simulink model "v2_4_debug3"  (R2017a)
settings: Solver=VariableStepAuto  StartTime=0.0  StopTime=50  RelTol=1e-3
values from neighbouring files (symbols this model uses):
  EbN0 = 6    [v2_4_debug1sI.m]    (also in v2_4_debug2sI.m; v2_4_debug3m.m; v2_4_randomm.m = 7; v2_4_randomm2.m)
  TracebackDepth = 64    [v2_4_debug1sI.m]    (also in v2_4_debug2sI.m; v2_4_debug3m.m; v2_4_randomm.m; v2_4_randomm2.m)
libraries: commblkintrlv2 x2, commchan3 x2, commdigbbndpm3 x1, commrandsrc3 x1, dspquant2 x1, commsink2 x1
settings Model: Creator=DELL  LastModifiedBy=DELL

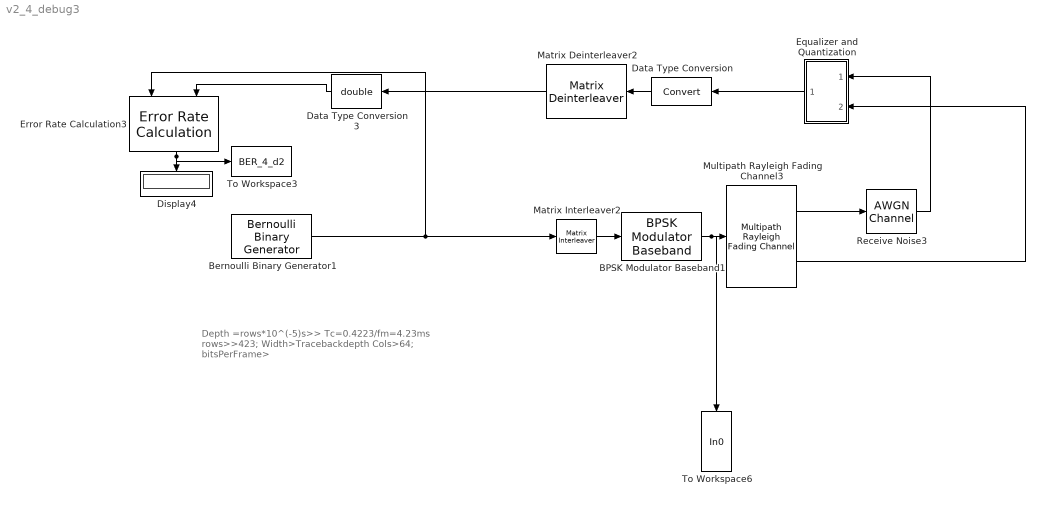
== system v2_4_debug3 ==
  note: Depth =rows*10^(-5)s>> Tc=0.4223/fm=4.23ms
      | 	rows>>423;
      |
      | Width>Tracebackdepth
      | 	Cols>64;
      |
      | bitsPerFrame>
  BPSK Modulator Baseband1 : commdigbbndpm3/BPSK Modulator Baseband  Ph=0  outDtype=double  outWordLen=16  outUDDataType=sfix(16)  outFracLenMode=Best precision  outFracLen=15  outDataTypeStr=double  outLastDataTypeStr=double
  Bernoulli Binary Generator1 : commrandsrc3/Bernoulli Binary Generator  ProbabilityOfZero=0.5  SeedSource=Auto  Seed=0  SampleTime=1e-5  SamplesPerFrame=SamplesPerFrame  OutputDataType=double  SimulateUsing=Interpreted execution
  Data Type Conversion : DataTypeConversion  SaturateOnIntegerOverflow=on  RndMeth=Zero
  Data Type Conversion3 : DataTypeConversion  OutDataTypeStr=double
  Display4 : Display
  Equalizer and Quantization : Subsystem
  Error Rate Calculation3 : commsink2/Error Rate Calculation  N=TracebackDepth  st_delay=0  cp_mode=Entire frame  subframe=[]  PMode=Port  WsName=ErrorVec  RsMode2=off  stop=off  numErr=100  maxBits=1e6
  Matrix Deinterleaver2 : commblkintrlv2/Matrix Deinterleaver  Nrows=Rows  Ncols=Cols
      settings: SourceProductName=Communications System Toolbox  SourceProductBaseCode=CM
  Matrix Interleaver2 : commblkintrlv2/Matrix Interleaver  Nrows=Rows  Ncols=Cols
      settings: SourceProductName=Communications System Toolbox  SourceProductBaseCode=CM
  Multipath Rayleigh Fading Channel3 : commchan3/Multipath Rayleigh Fading Channel  maxDopplerShift=100  spectrumType=Jakes  sigmaGaussian=1/sqrt(2)  coeffRounded=[1 -1.72 0.785]  freqMinMaxRJakes=[0 1]  freqMinMaxAJakes=[0 1]  sigmaGaussian1=1/sqrt(2)  sigmaGaussian2=1/sqrt(2)  centerFreqGaussian1=0.0  centerFreqGaussian2=0.0  gainGaussian1=0.5  gainGaussian2=0.5  coeffBell=9  dopplerSpectrum=doppler.jakes  pathDelays=0  avgPathGaindB=2  normalizePathGains=on  seed=12345  enableProbe=0  openVisAtStart=off  outPathGains=on  outDelay=off
      settings: SourceProductName=Communications System Toolbox  SourceProductBaseCode=CM
  Receive Noise3 : commchan3/AWGN Channel  InputProcessing=Columns as channels (frame based)  seed=188  noiseMode="Signal to noise ratio  (Eb/No)"  EbNodB=EbN0  EsNodB=EbNo  SNRdB=50  bitsPerSym=1  Ps=1  Tsym=1e-5  variance=1
  To Workspace3 : ToWorkspace  VariableName=BER_4_d2  SampleTime=-1
      settings: MaxDataPoints=1
  To Workspace6 : ToWorkspace  VariableName=In0  SampleTime=-1
      settings: MaxDataPoints=1
  wires:
  BPSK Modulator Baseband1/1 -> To Workspace6/1, Multipath Rayleigh Fading Channel3/1
  Error Rate Calculation3/1 -> To Workspace3/1, Display4/1
  Multipath Rayleigh Fading Channel3/1 -> Receive Noise3/1
  Data Type Conversion3/1 -> Error Rate Calculation3/2
  Matrix Interleaver2/1 -> BPSK Modulator Baseband1/1
  Bernoulli Binary Generator1/1 -> Matrix Interleaver2/1, Error Rate Calculation3/1
  Matrix Deinterleaver2/1 -> Data Type Conversion3/1
  Data Type Conversion/1 -> Matrix Deinterleaver2/1
  Receive Noise3/1 -> Equalizer and Quantization/1(In1)
  Multipath Rayleigh Fading Channel3/2 -> Equalizer and Quantization/2(In2)
  Equalizer and Quantization/1(Out1) -> Data Type Conversion/1

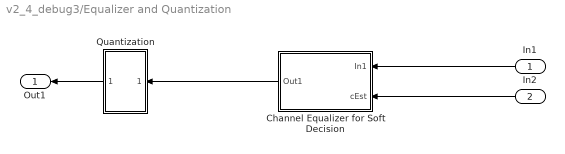
== system v2_4_debug3/Equalizer and Quantization ==
  In1 : Inport
  In2 : Inport  Port=2
  Channel Equalizer for Soft Decision : Subsystem
      mask Display:
      | disp('Equalizer');
      | port_label('input', 2, 'cEst');
  Quantization : Subsystem  Tag=UniformEncoder
  Out1 : Outport
  wires:
  In2/1 -> Channel Equalizer for Soft Decision/2(cEst)
  In1/1 -> Channel Equalizer for Soft Decision/1(In1)
  Channel Equalizer for Soft Decision/1(Out1) -> Quantization/1(In1)
  Quantization/1(Out1) -> Out1/1

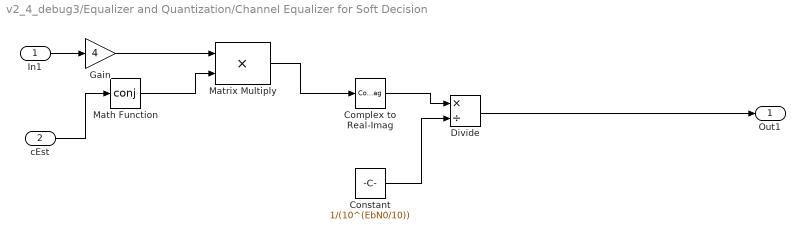
== system v2_4_debug3/Equalizer and Quantization/Channel Equalizer for Soft Decision ==
  In1 : Inport
  cEst : Inport  Port=2
  Complex to Real-Imag : ComplexToRealImag  Output=Real
  Constant : Constant  Value=1/(10^(EbN0/10))
  Divide : Product  Inputs=*/
  Gain : Gain  Gain=4
  Math Function : Math  Operator=conj  SaturateOnIntegerOverflow=on
  Matrix Multiply : Product
  Out1 : Outport
  wires:
  In1/1 -> Gain/1
  cEst/1 -> Math Function/1
  Matrix Multiply/1 -> Complex to Real-Imag/1
  Divide/1 -> Out1/1
  Math Function/1 -> Matrix Multiply/2
  Gain/1 -> Matrix Multiply/1
  Constant/1 -> Divide/2
  Complex to Real-Imag/1 -> Divide/1

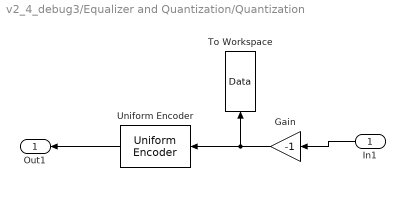
== system v2_4_debug3/Equalizer and Quantization/Quantization ==
  In1 : Inport
  Gain : Gain  Gain=-1  SaturateOnIntegerOverflow=on  OutDataTypeStr=Inherit: Same as input  ParamDataTypeStr=Inherit: Same as input
  To Workspace : ToWorkspace  VariableName=Data  SampleTime=-1
      settings: MaxDataPoints=1
  Uniform Encoder : dspquant2/Uniform Encoder  peak=peak  bits=8  otype=Unsigned integer
      settings: SourceProductName=DSP System Toolbox
  Out1 : Outport
  wires:
  Uniform Encoder/1 -> Out1/1
  Gain/1 -> To Workspace/1, Uniform Encoder/1
  In1/1 -> Gain/1
